simulink model "motor_pi"  (R2018b)
settings: Solver=FixedStepAuto  StartTime=0.0  StopTime=20  FixedStep=0.01  RelTol=1e-3
undefined symbols (not defined in the file): Ki_l, Ki_r, Kl, Kp_l, Kp_r, Kr, Ll, Lr, Ti_l, Ti_r, Tl, Tr, Ts
libraries: simulink x4
settings Model: Creator=kshat  LastModifiedBy=m152069
settings OptimizationCC: DefaultParameterBehavior=Inlined  UseDivisionForNetSlopeComputation=on  UseFloatMulNetSlope=on  InlineInvariantSignals=on  PassReuseOutputArgsAs=Individual arguments  ZeroExternalMemoryAtStartup=off  ZeroInternalMemoryAtStartup=off  NoFixptDivByZeroProtection=on  EfficientFloat2IntCast=on  LifeSpan=1  OptimizeBlockOrder=speed  DifferentSizesBufferReuse=on
settings DebuggingCC: ParameterTunabilityLossMsg=error  LibraryContextMissingDiagnostic=none
settings HardwareCC: ProdBitPerPointer=32  ProdBitPerSizeT=32  ProdBitPerPtrDiffT=32  ProdLargestAtomicInteger=Long  ProdWordSize=32  ProdLongLongMode=on  ProdHWDeviceType=ARM Compatible->ARM 9
settings SFSimCC: SimUseLocalCustomCode=off  MATLABDynamicMemAlloc=off
settings RTWCC: SystemTargetFile=ert.tlc  TemplateMakefile=ert_default_tmf  GenerateReport=on  RTWUseLocalCustomCode=off  IncludeHyperlinkInReport=on  LaunchReport=on  TargetLang=C++  GenerateTraceInfo=on  GenerateTraceReport=on  GenerateTraceReportSl=on  GenerateTraceReportSf=on  GenerateTraceReportEml=on
settings CodeAppCC: ForceParamTrailComments=on  IgnoreCustomStorageClasses=off  OperatorAnnotations=on  SimulinkDataObjDesc=on  SFDataObjDesc=on  CustomSymbolStrGlobalVar=rt$N$M  CustomSymbolStrType=$N$M  CustomSymbolStrFcn=$N$M$F  CustomSymbolStrMacro=$N$M  InsertBlockDesc=on
settings ERTTargetCC: TargetLangStandard=C++03 (ISO)  GenerateSampleERTMain=on  IncludeMdlTerminateFcn=off  CombineSignalStateStructs=on  MultiInstanceERTCode=on  CodeInterfacePackaging=C++ class  SupportComplex=off  SupportContinuousTime=on  InlinedParameterPlacement=NonHierarchical  RootIOFormat=Structure reference  ERTCustomFileTemplate=example_file_process.tlc  ERTFilePackagingFormat=CompactWithDataFile

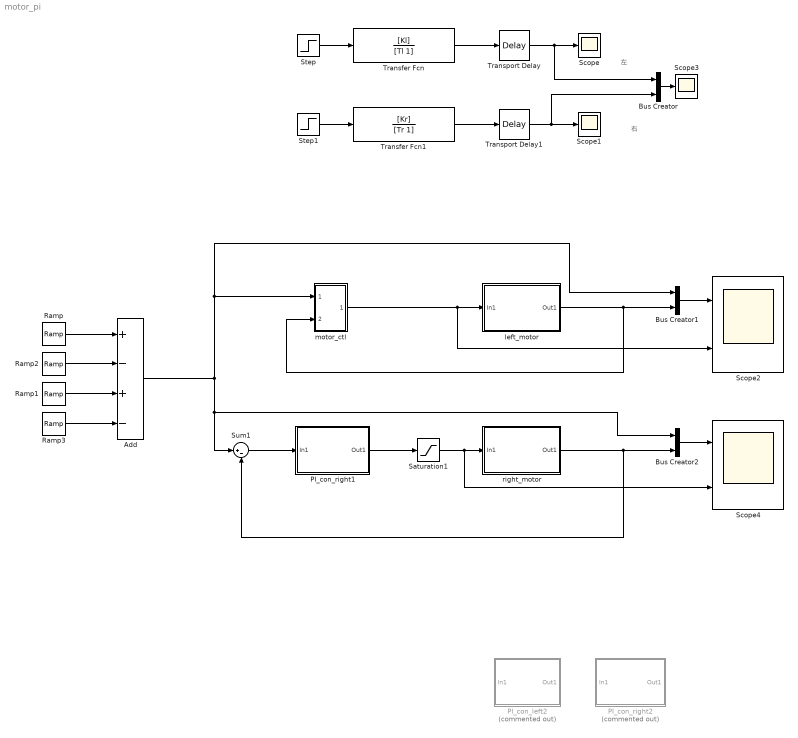
== system motor_pi ==
  note: 右
  note: 左
  Add : Sum  Inputs=+-+-
  Bus Creator : BusCreator  Inputs=2
  Bus Creator1 : BusCreator  Inputs=2
  Bus Creator2 : BusCreator  Inputs=2
  PI_con_left2 : Subsystem  Commented=on
  PI_con_right1 : Subsystem
  PI_con_right2 : Subsystem  Commented=on
  Ramp : simulink/Sources/Ramp  slope=200  start=2  InitialOutput=0
  Ramp1 : simulink/Sources/Ramp  slope=-200  start=14  InitialOutput=0
  Ramp2 : simulink/Sources/Ramp  slope=200  start=4  InitialOutput=0
  Ramp3 : simulink/Sources/Ramp  slope=-200  start=16  InitialOutput=0
  Saturation1 : Saturate  UpperLimit=100  LowerLimit=0
  Scope : Scope
  Scope1 : Scope
  Scope2 : Scope  NumInputPorts=2
  Scope3 : Scope
  Scope4 : Scope  NumInputPorts=2
  Step : Step  Time=0  After=100  SampleTime=0
  Step1 : Step  Time=0  After=100  SampleTime=0
  Sum1 : Sum  Inputs=|+-
  Transfer Fcn : TransferFcn  Numerator=[Kl]  Denominator=[Tl 1]
  Transfer Fcn1 : TransferFcn  Numerator=[Kr]  Denominator=[Tr 1]
  Transport Delay : TransportDelay  DelayTime=Ll
  Transport Delay1 : TransportDelay  DelayTime=Lr
  left_motor : Subsystem
  motor_ctl : Subsystem  TreatAsAtomicUnit=on
  right_motor : Subsystem
  wires:
  Step/1 -> Transfer Fcn/1
  Transfer Fcn/1 -> Transport Delay/1
  Transport Delay/1 -> Bus Creator/1, Scope/1
  Transfer Fcn1/1 -> Transport Delay1/1
  Step1/1 -> Transfer Fcn1/1
  Transport Delay1/1 -> Bus Creator/2, Scope1/1
  Add/1 -> Bus Creator2/1, Sum1/1, motor_ctl/1(In1), Bus Creator1/1
  Bus Creator/1 -> Scope3/1
  left_motor/1(Out1) -> motor_ctl/2(In2), Bus Creator1/2
  PI_con_right1/1(Out1) -> Saturation1/1
  right_motor/1(Out1) -> Sum1/2, Bus Creator2/2
  Sum1/1 -> PI_con_right1/1(In1)
  Bus Creator1/1 -> Scope2/1
  Bus Creator2/1 -> Scope4/1
  Saturation1/1 -> Scope4/2, right_motor/1(In1)
  Ramp/1 -> Add/1
  Ramp2/1 -> Add/2
  Ramp1/1 -> Add/3
  Ramp3/1 -> Add/4
  motor_ctl/1(Out1) -> Scope2/2, left_motor/1(In1)

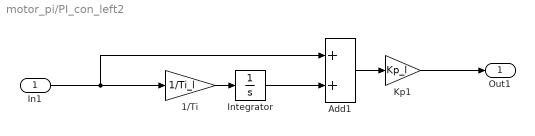
== system motor_pi/PI_con_left2 ==
  In1 : Inport
  1/Ti : Gain  Gain=1/Ti_l
  Add1 : Sum
  Integrator : Integrator
  Kp1 : Gain  Gain=Kp_l
  Out1 : Outport
  wires:
  Integrator/1 -> Add1/2
  In1/1 -> Add1/1, 1/Ti/1
  Kp1/1 -> Out1/1
  1/Ti/1 -> Integrator/1
  Add1/1 -> Kp1/1

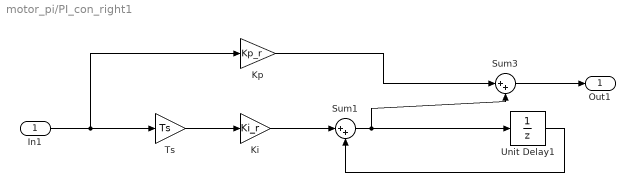
== system motor_pi/PI_con_right1 ==
  In1 : Inport
  Ki : Gain  Gain=Ki_r
  Kp : Gain  Gain=Kp_r
  Sum1 : Sum  Inputs=|++
  Sum3 : Sum  Inputs=|++
  Ts : Gain  Gain=Ts
  Unit Delay1 : UnitDelay  SampleTime=-1
  Out1 : Outport
  wires:
  Sum3/1 -> Out1/1
  Sum1/1 -> Unit Delay1/1, Sum3/2
  Ki/1 -> Sum1/1
  Kp/1 -> Sum3/1
  Ts/1 -> Ki/1
  Unit Delay1/1 -> Sum1/2
  In1/1 -> Kp/1, Ts/1

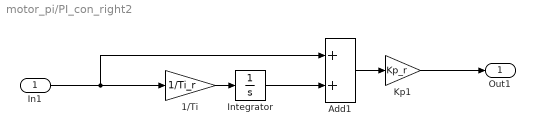
== system motor_pi/PI_con_right2 ==
  In1 : Inport
  1/Ti : Gain  Gain=1/Ti_r
  Add1 : Sum
  Integrator : Integrator
  Kp1 : Gain  Gain=Kp_r
  Out1 : Outport
  wires:
  Add1/1 -> Kp1/1
  1/Ti/1 -> Integrator/1
  Kp1/1 -> Out1/1
  In1/1 -> 1/Ti/1, Add1/1
  Integrator/1 -> Add1/2

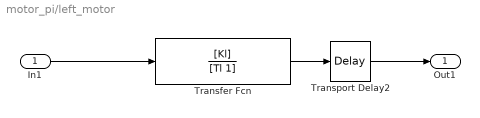
== system motor_pi/left_motor ==
  In1 : Inport
  Transfer Fcn : TransferFcn  Numerator=[Kl]  Denominator=[Tl 1]
  Transport Delay2 : TransportDelay  DelayTime=Ll
  Out1 : Outport
  wires:
  Transfer Fcn/1 -> Transport Delay2/1
  In1/1 -> Transfer Fcn/1
  Transport Delay2/1 -> Out1/1

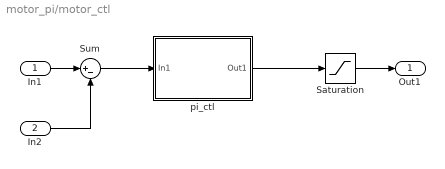
== system motor_pi/motor_ctl ==
  In1 : Inport
  In2 : Inport  Port=2
  Saturation : Saturate  UpperLimit=100  LowerLimit=0
  Sum : Sum  Inputs=|+-
  pi_ctl : Subsystem
  Out1 : Outport
  wires:
  In1/1 -> Sum/1
  Sum/1 -> pi_ctl/1(In1)
  pi_ctl/1(Out1) -> Saturation/1
  In2/1 -> Sum/2
  Saturation/1 -> Out1/1

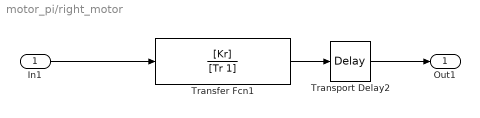
== system motor_pi/right_motor ==
  In1 : Inport
  Transfer Fcn1 : TransferFcn  Numerator=[Kr]  Denominator=[Tr 1]
  Transport Delay2 : TransportDelay  DelayTime=Lr
  Out1 : Outport
  wires:
  Transport Delay2/1 -> Out1/1
  In1/1 -> Transfer Fcn1/1
  Transfer Fcn1/1 -> Transport Delay2/1

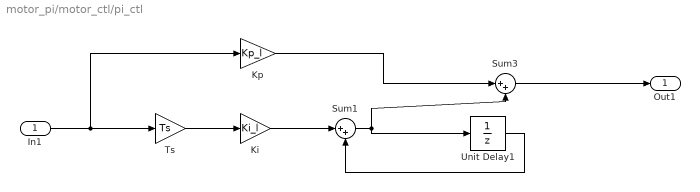
== system motor_pi/motor_ctl/pi_ctl ==
  In1 : Inport
  Ki : Gain  Gain=Ki_l
  Kp : Gain  Gain=Kp_l
  Sum1 : Sum  Inputs=|++
  Sum3 : Sum  Inputs=|++
  Ts : Gain  Gain=Ts
  Unit Delay1 : UnitDelay  SampleTime=-1
  Out1 : Outport
  wires:
  In1/1 -> Ts/1, Kp/1
  Unit Delay1/1 -> Sum1/2
  Ts/1 -> Ki/1
  Kp/1 -> Sum3/1
  Ki/1 -> Sum1/1
  Sum1/1 -> Sum3/2, Unit Delay1/1
  Sum3/1 -> Out1/1
